simulink model "Xe_chay_diem_target_nhap_theo_quy_dao_R"  (R2021b)
settings: Solver=VariableStepAuto  StartTime=1  StopTime=30  RelTol=1e-3
settings Model: Creator=HL_1810  LastModifiedBy=ASUS

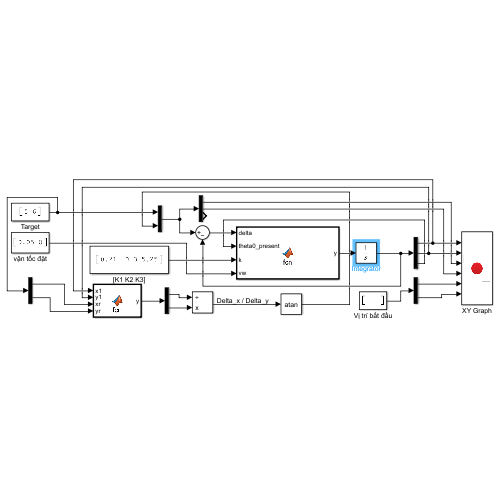
[thumbnail: Simulink's stored preview of the top-level diagram]
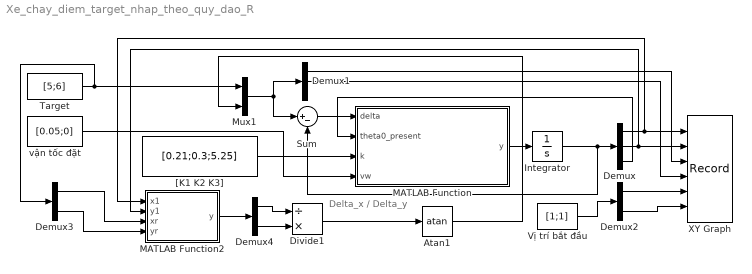
== system Xe_chay_diem_target_nhap_theo_quy_dao_R ==
  note: Delta_x / Delta_y
  Atan1 : Trigonometry  Operator=atan
  Demux : Demux  Outputs=3
  Demux1 : Demux  Outputs=3
  Demux2 : Demux  Outputs=2
  Demux3 : Demux  Outputs=2
  Demux4 : Demux  Outputs=2
  Divide1 : Product  Inputs=/*
  Integrator : Integrator  InitialCondition=[1;1;pi/6]
  MATLAB Function : MATLAB Function  TreatAsAtomicUnit=on
  MATLAB Function2 : MATLAB Function  TreatAsAtomicUnit=on
  Mux1 : Mux  Inputs=2
  Sum : Sum  Inputs=|+-
  Target : Constant  Value=[5;6]
  Vị trí bắt đầu : Constant  Value=[1;1]
  XY Graph : Record  FileSettingsInternal="{\"entries\":[{\"content\":{\"excelSettings\":{\"content\":{},\"type\":\"Streamout.ExcelSettings\"}},\"type\":\"Streamout.FileSettingStorage\",\"uuid\":\"d778f314-aa44-472d-93c3-3ca5c424359a\"}],\"packageUris\":[\"http://schema.mathworks.com/mf0/streamout_blocks/R2020a\"],\"version\":\"1.0\"}"  Layout=[1 1]  SignalsInternal="{\"entries\":[{\"content\":{\"signals\":[{\"content\":{\"blockPath\":[\"Xe_chay_diem_target_nhap_theo_quy_dao_R/XY Graph\"],\"channel\":[],\"dimensions\":[1],\"domain\":\"Xe_chay_diem_target_nhap_theo_quy_dao_R/XY Graph\",\"lineColor\":\"#edb120\",\"plots\":[1],\"port\":1,\"sid\":[\"\"],\"signalID\":2169,\"signalName\":\"Demux:1\"},\"type\":\"RecordBlkView.Signal\",\"uuid\":\"b1771882-ce94-4be2-857d-a5152cf5ea78\"},{\"content\":{\"blockPath\":[\"Xe_chay_diem_target_nhap_theo_quy_dao_R/XY Graph\"],\"channel\":[],\"dimensions\":[1],\"domain\":\"Xe_chay_diem_target_nhap_theo_quy_dao_R/XY Graph\",\"lineColor\":\"#7e2f8e\",\"plots\":[1],\"port\":2,\"sid\":[\"\"],\"signalID\":2173,\"signalName\":\"Demux:2\"},\"type\":\"RecordBlkView.Signal\",\"uuid\":\"e838813a-a239-4284-9f85-4624bd99f148\"},{\"content\":{\"blockPath\":[\"Xe_chay_diem_target_nhap_theo_quy_dao_R/XY Graph\"],\"channel\":[],\"dimensions\":[1],\"domain\":\"Xe_chay_diem_target_nhap_theo_quy_dao_R/XY Graph\",\"lineColor\":\"#77ac30\",\"plots\":[1],\"port\":3,\"sid\":[\"\"],\"signalID\":2177,\"signalName\":\"Demux1:1\"},\"type\":\"RecordBlkView.Signal\",\"uuid\":\"e12a6854-baf0-470c-9932-345a9d7901ba\"},{\"content\":{\"blockPath\":[\"Xe_chay_diem_target_nhap_theo_quy_dao_R/XY Graph\"],\"channel\":[],\"dimensions\":[1],\"domain\":\"Xe_chay_diem_target_nhap_theo_quy_dao_R/XY Graph\",\"lineColor\":\"#4dbeee\",\"plots\":[1],\"port\":4,\"sid\":[\"\"],\"signalID\":2181,\"signalName\":\"Demux1:2\"},\"type\":\"RecordBlkView.Signal\",\"uuid\":\"46057b67-2117-4207-87f3-2c33b01df444\"},{\"content\":{\"blockPath\":[\"Xe_chay_diem_target_nhap_theo_quy_dao_R/XY Graph\"],\"channel\":[],\"dimensions\":[1],\"domain\":\"Xe_chay_diem_target_nhap_theo_quy_dao_R/XY Graph\",\"lineColor\":\"#a2142f\",\"plots\":[1],\"port\":5,\"sid\":[\"\"],\"signalID\":2185,\"signalName\":\"Demux2:1\"},\"type\":\"RecordBlkView.Signal\",\"uuid\":\"7f1cb56e-e097-4c3a-a5c3-6c0dc9702bc0\"},{\"content\":{\"blockPath\":[\"Xe_chay_diem_target_nhap_theo_quy_dao_R/XY Graph\"],\"channel\":[],\"dimensions\":[1],\"domain\":\"Xe_chay_diem_target_nhap_theo_quy_dao_R/XY Graph\",\"lineColor\":\"#139fff\",\"plots\":[1],\"port\":6,\"sid\":[\"\"],\"signalID\":2189,\"signalName\":\"Demux2:2\"},\"type\":\"RecordBlkView.Signal\",\"uuid\":\"8f8b8fb7-040b-47e3-87e7-4127c94107bd\"}]},\"type\":\"RecordBlkView.InputSignals\",\"uuid\":\"b5f76768-6cfe-49b0-9edb-da571d3d4d41\"}],\"packageUris\":[\"http://schema.mathworks.com/mf0/streamout_blocks/R2020a\"],\"version\":\"1.0\"}"  VisualizationBindings="{\"xyplotplugin\":{\"info\":[{\"series\":[{\"bindingParametersList\":[{\"parameter\":\"X-Axis\",\"signalID\":2185,\"signalName\":\"Demux2:1\"},{\"parameter\":\"Y-Axis\",\"signalID\":2189,\"signalName\":\"Demux2:2\"}],\"seriesID\":57161},{\"bindingParametersList\":[{\"parameter\":\"X-Axis\",\"signalID\":2177,\"signalName\":\"Demux1:1\"},{\"parameter\":\"Y-Axis\",\"signalID\":2181,\"signalName\":\"Demux1:2\"}],\"seriesID\":5755},{\"bindingParametersList\":[{\"parameter\":\"Y-Axis\",\"signalID\":2173,\"signalName\":\"Demux:2\"},{\"parameter\":\"X-Axis\",\"signalID\":2169,\"signalName\":\"Demux:1\"}],\"seriesID\":6466}],\"subplotID\":1},{\"series\":[],\"subplotID\":2}]}}"  CompatibilityTag=XY
  "[K1 K2 K3]" : Constant  Value=[0.21;0.3;5.25]
  vận tốc đặt : Constant  Value=[0.05;0]
  wires:
  Integrator/1 -> Sum/2, Demux/1
  Demux/3 -> MATLAB Function/2(theta0_present)
  Sum/1 -> MATLAB Function/1(delta)
  Demux1/2 -> XY Graph/4
  Demux/1 -> MATLAB Function2/1(x1), XY Graph/1
  Demux/2 -> MATLAB Function2/2(y1), XY Graph/2
  "[K1 K2 K3]"/1 -> MATLAB Function/3(k)
  Demux1/1 -> XY Graph/3
  MATLAB Function/1(y) -> Integrator/1
  vận tốc đặt/1 -> MATLAB Function/4(vw)
  Target/1 -> Demux3/1, Mux1/1
  Demux3/1 -> MATLAB Function2/3(xr)
  Demux3/2 -> MATLAB Function2/4(yr)
  MATLAB Function2/1(y) -> Demux4/1
  Divide1/1 -> Atan1/1
  Atan1/1 -> Mux1/2
  Mux1/1 -> Demux1/1, Sum/1
  Vị trí bắt đầu/1 -> Demux2/1
  Demux2/1 -> XY Graph/5
  Demux2/2 -> XY Graph/6
  Demux4/2 -> Divide1/2
  Demux4/1 -> Divide1/1

== matlab function Xe_chay_diem_target_nhap_theo_quy_dao_R/MATLAB Function ==
  data: delta input; y output; theta0_present input; k input; vw input
function y = fcn(delta,theta0_present,k,vw)
%#codegen
A=[cos(theta0_present)   sin(theta0_present) 0;
    -sin(theta0_present) cos(theta0_present) 0;
    0                    0                    1];
e=A*delta;
V_c=[vw(1)*cos(e(3))+k(1)*e(1);
    vw(2)+k(2)*vw(1)*e(2)+k(3)*vw(1)*sin(e(3))];
Matrix=[cos(theta0_present) 0;
        sin(theta0_present) 0;
        0                   1];
u=Matrix*V_c;
y = u;

== matlab function Xe_chay_diem_target_nhap_theo_quy_dao_R/MATLAB Function2 ==
  data: x1 input; y output; y1 input; xr input; yr input
function y = fcn(x1,y1,xr,yr)
%#codegen
x_delta=xr-x1;
y_delta=yr-y1;
u=[x_delta;y_delta]
y = u;
